simulink model "DrvStFtCtrl"  (R2018b)
settings: Solver=FixedStepDiscrete  StartTime=0.0  StopTime=10.0  FixedStep=0.01  RelTol=1e-3
undefined symbols (not defined in the file or in its folder): KeSMSuMdMotFinshdTm_Val, KeSMSuMdRetryTm1_Val, KeSMSuModeReqDurgTm_Val, KeSMSwDrvStFtEnTrigBitMask_Val
libraries: StCtrlLib x1
settings Model: Creator=sn2xws  LastModifiedBy=sn2xws
settings DataIOCC: SaveFormat=StructureWithTime
settings OptimizationCC: DefaultParameterBehavior=Inlined  EnhancedBackFolding=on  PassReuseOutputArgsAs=Individual arguments  ZeroExternalMemoryAtStartup=off  ZeroInternalMemoryAtStartup=off  OptimizeBlockOrder=speed  DifferentSizesBufferReuse=on  OptimizationCustomize=off
settings DebuggingCC: ParameterTunabilityLossMsg=error
settings ModelReferenceCC: ModelReferenceNumInstancesAllowed=Single
settings SFSimCC: MATLABDynamicMemAlloc=off
settings RTWCC: SystemTargetFile=autosar.tlc  GenCodeOnly=on  TemplateMakefile=ert_default_tmf  Description=AUTOSAR  GenerateReport=on  IncludeHyperlinkInReport=on  LaunchReport=on  GenerateTraceInfo=on  GenerateTraceReport=on  GenerateTraceReportSl=on  GenerateTraceReportSf=on  GenerateTraceReportEml=on  GenerateCodeMetricsReport=on
settings CodeAppCC: ForceParamTrailComments=on  IgnoreCustomStorageClasses=off  OperatorAnnotations=on  SimulinkDataObjDesc=on  SFDataObjDesc=on  InsertBlockDesc=on
settings STFCustomTargetCC: TargetLangStandard=C99 (ISO)  MultiwordLength=256  ParMdlRefBuildCompliant=on  CompOptLevelCompliant=on  IncludeMdlTerminateFcn=off  CombineOutputUpdateFcns=on  SuppressErrorStatus=on  ERTCustomFileBanners=on  SupportNonFinite=off  SupportComplex=off  SupportContinuousTime=off  SupportNonInlinedSFcns=off  RemoveResetFunc=on  MATLABClassNameForMDSCustomization=Simulink.SoftwareTarget.ERTCustomization  AutosarCompliant=on  UseToolchainInfoCompliant=on  LookupTableObjectStructAxisOrder=2,1,3,4,...  LUTObjectStructOrderEvenSpacing=Size,Table,Breakpoints  SystemTargetFile=autosar.tlc
settings ERTTargetCC: TargetLangStandard=C99 (ISO)  ConcurrentExecutionCompliant=off  IncludeMdlTerminateFcn=off  SuppressErrorStatus=on  SupportNonFinite=off  SupportComplex=off  ModelStepFunctionPrototypeControlCompliant=off  CPPClassGenCompliant=off  AutosarCompliant=on  LookupTableObjectStructAxisOrder=2,1,3,4,...  LUTObjectStructOrderEvenSpacing=Size,Table,Breakpoints  InlinedParameterPlacement=NonHierarchical  ERTCustomFileTemplate=example_file_process.tlc  ERTFilePackagingFormat=Compact

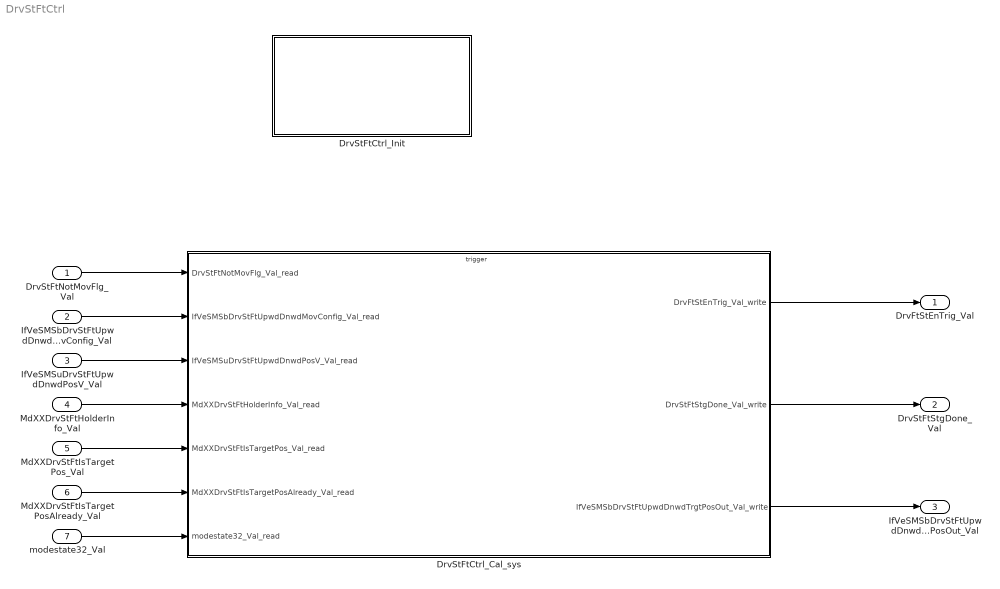
== system DrvStFtCtrl ==
  DrvStFtNotMovFlg_Val : Inport  OutDataTypeStr=boolean  PortDimensions=1
  IfVeSMSbDrvStFtUpwdDnwdMovConfig_Val : Inport  Port=2  OutDataTypeStr=boolean  PortDimensions=1
  IfVeSMSuDrvStFtUpwdDnwdPosV_Val : Inport  Port=3  OutDataTypeStr=boolean  PortDimensions=1
  MdXXDrvStFtHolderInfo_Val : Inport  Port=4  OutDataTypeStr=uint32  PortDimensions=1
  MdXXDrvStFtIsTargetPos_Val : Inport  Port=5  OutDataTypeStr=uint32  PortDimensions=1
  MdXXDrvStFtIsTargetPosAlready_Val : Inport  Port=6  OutDataTypeStr=uint32  PortDimensions=1
  modestate32_Val : Inport  Port=7  OutDataTypeStr=uint32  PortDimensions=1
  DrvStFtCtrl_Cal_sys : Subsystem
  DrvStFtCtrl_Init : Subsystem
  DrvFtStEnTrig_Val : Outport  OutDataTypeStr=boolean  PortDimensions=1
  DrvStFtStgDone_Val : Outport  Port=2  OutDataTypeStr=boolean  PortDimensions=1
  IfVeSMSbDrvStFtUpwdDnwdTrgtPosOut_Val : Outport  Port=3  OutDataTypeStr=boolean  PortDimensions=1
  wires:
  DrvStFtCtrl_Cal_sys/1(DrvFtStEnTrig_Val_write) -> DrvFtStEnTrig_Val/1
  DrvStFtCtrl_Cal_sys/2(DrvStFtStgDone_Val_write) -> DrvStFtStgDone_Val/1
  DrvStFtCtrl_Cal_sys/3(IfVeSMSbDrvStFtUpwdDnwdTrgtPosOut_Val_write) -> IfVeSMSbDrvStFtUpwdDnwdTrgtPosOut_Val/1
  DrvStFtNotMovFlg_Val/1 -> DrvStFtCtrl_Cal_sys/1(DrvStFtNotMovFlg_Val_read)
  IfVeSMSbDrvStFtUpwdDnwdMovConfig_Val/1 -> DrvStFtCtrl_Cal_sys/2(IfVeSMSbDrvStFtUpwdDnwdMovConfig_Val_read)
  IfVeSMSuDrvStFtUpwdDnwdPosV_Val/1 -> DrvStFtCtrl_Cal_sys/3(IfVeSMSuDrvStFtUpwdDnwdPosV_Val_read)
  MdXXDrvStFtHolderInfo_Val/1 -> DrvStFtCtrl_Cal_sys/4(MdXXDrvStFtHolderInfo_Val_read)
  MdXXDrvStFtIsTargetPos_Val/1 -> DrvStFtCtrl_Cal_sys/5(MdXXDrvStFtIsTargetPos_Val_read)
  MdXXDrvStFtIsTargetPosAlready_Val/1 -> DrvStFtCtrl_Cal_sys/6(MdXXDrvStFtIsTargetPosAlready_Val_read)
  modestate32_Val/1 -> DrvStFtCtrl_Cal_sys/7(modestate32_Val_read)

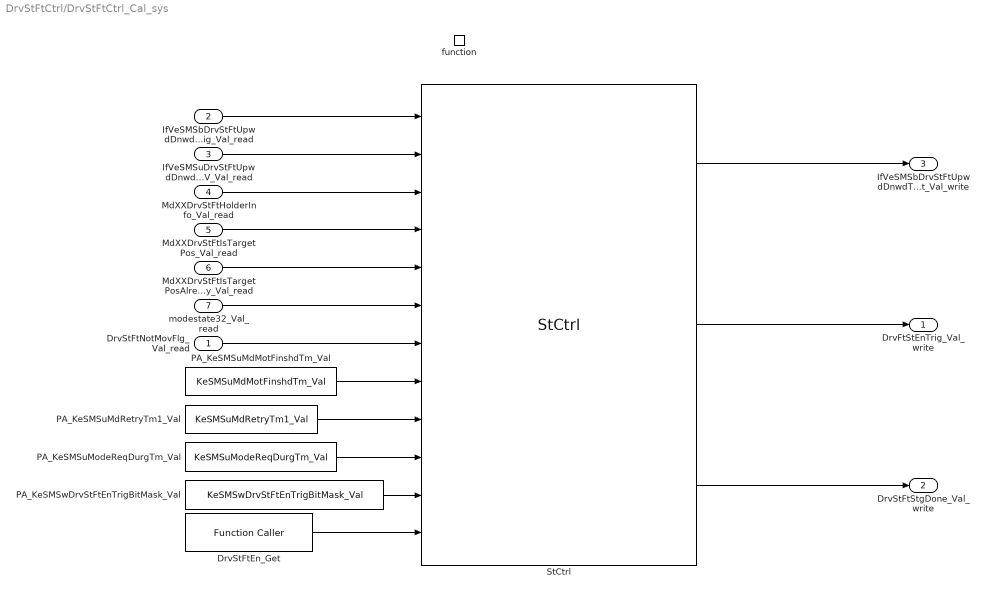
== system DrvStFtCtrl/DrvStFtCtrl_Cal_sys ==
  DrvStFtNotMovFlg_Val_read : Inport
  IfVeSMSbDrvStFtUpwdDnwdMovConfig_Val_read : Inport  Port=2
  IfVeSMSuDrvStFtUpwdDnwdPosV_Val_read : Inport  Port=3
  MdXXDrvStFtHolderInfo_Val_read : Inport  Port=4
  MdXXDrvStFtIsTargetPos_Val_read : Inport  Port=5
  MdXXDrvStFtIsTargetPosAlready_Val_read : Inport  Port=6
  modestate32_Val_read : Inport  Port=7
  function : TriggerPort  TriggerType=function-call  IsSimulinkFunction=on  FunctionName=DrvStFtCtrl_Cal  VariantControl=(inherit)
  DrvStFtEn_Get : FunctionCaller  FunctionPrototype=data = DrvStFtEn_Get()  OutputArgumentSpecifications=uint32(1)
  PA_KeSMSuMdMotFinshdTm_Val : Constant  Value=KeSMSuMdMotFinshdTm_Val
  PA_KeSMSuMdRetryTm1_Val : Constant  Value=KeSMSuMdRetryTm1_Val
  PA_KeSMSuModeReqDurgTm_Val : Constant  Value=KeSMSuModeReqDurgTm_Val
  PA_KeSMSwDrvStFtEnTrigBitMask_Val : Constant  Value=KeSMSwDrvStFtEnTrigBitMask_Val
  StCtrl : StCtrlLib/StCtrl  SystemSampleTime=-1
  DrvFtStEnTrig_Val_write : Outport
      settings: EnsureOutportIsVirtual=on
  DrvStFtStgDone_Val_write : Outport  Port=2
      settings: EnsureOutportIsVirtual=on
  IfVeSMSbDrvStFtUpwdDnwdTrgtPosOut_Val_write : Outport  Port=3
      settings: EnsureOutportIsVirtual=on
  wires:
  DrvStFtEn_Get/1 -> StCtrl/12
  PA_KeSMSuMdMotFinshdTm_Val/1 -> StCtrl/8
  PA_KeSMSuMdRetryTm1_Val/1 -> StCtrl/9
  PA_KeSMSuModeReqDurgTm_Val/1 -> StCtrl/10
  StCtrl/2 -> DrvFtStEnTrig_Val_write/1
  StCtrl/3 -> DrvStFtStgDone_Val_write/1
  StCtrl/1 -> IfVeSMSbDrvStFtUpwdDnwdTrgtPosOut_Val_write/1
  DrvStFtNotMovFlg_Val_read/1 -> StCtrl/7
  IfVeSMSbDrvStFtUpwdDnwdMovConfig_Val_read/1 -> StCtrl/1
  IfVeSMSuDrvStFtUpwdDnwdPosV_Val_read/1 -> StCtrl/2
  MdXXDrvStFtHolderInfo_Val_read/1 -> StCtrl/3
  MdXXDrvStFtIsTargetPos_Val_read/1 -> StCtrl/4
  MdXXDrvStFtIsTargetPosAlready_Val_read/1 -> StCtrl/5
  modestate32_Val_read/1 -> StCtrl/6
  PA_KeSMSwDrvStFtEnTrigBitMask_Val/1 -> StCtrl/11

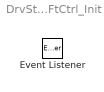
== system DrvStFtCtrl/DrvStFtCtrl_Init ==
  Event Listener : EventListener  EventName=reset
